simulink model "truck_suspen"  (R2020a)
settings: Solver=VariableStepAuto  StartTime=0.0  StopTime=100  RelTol=1e-3
settings Model: Creator=Shubham  LastModifiedBy=Shubham

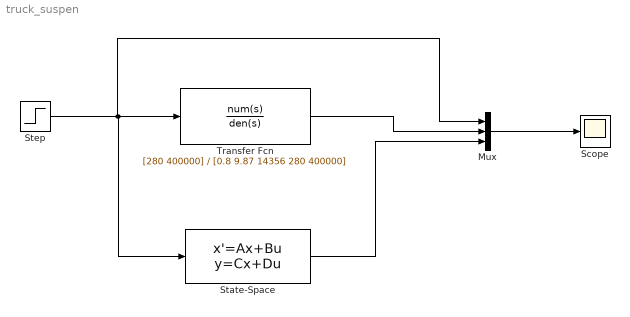
== system truck_suspen ==
  Mux : Mux  Inputs=3
  Scope : Scope
  State-Space : StateSpace  A=[-12.3375 -17945 -350 -500000;1 0 0 0;0 1 0 0;0 0 1 0]  B=[1;0;0;0]  C=[0,0,350,500000]  D=0  InitialCondition=0
  Step : Step  SampleTime=0
  Transfer Fcn : TransferFcn  Numerator=[280 400000]  Denominator=[0.8 9.87 14356 280 400000]
  wires:
  Step/1 -> Mux/1, State-Space/1, Transfer Fcn/1
  Mux/1 -> Scope/1
  State-Space/1 -> Mux/3
  Transfer Fcn/1 -> Mux/2
